simulink model "Aircraft6dof_V2"  (R2025b)
settings: Solver=ode4  StartTime=startTime  StopTime=A8.stopTime  FixedStep=stepTime  RelTol=1e-3  EnableMultiTasking=on
values from neighbouring files (symbols this model uses):
  A8 = struct()    [Setup_A8_master.m]
  InitAtt = InitAtt_deg * deg2rad    [Setup_A8_master.m]
  K_lqr_cmd = DeMixMatrix_val * K_lqr    [Design_LQR_Controller.m]
  n_p1 = axis_body    [Setup_A8_master.m]
undefined symbols (not defined in the file or in its folder): a0_s2, a0_s3, a0_s4, a0_s5, AR_s2, AR_s3, AR_s4, AR_s5, ARvecP1, Att_Trim, c_s2, c_s3, c_s4, c_s5, CD0_s2, CD0_s3, CD0_s4, CD0_s5, CDa_s2, CDa_s3, CDa_s4, CDa_s5, CL0_s2, CL0_s3, CL0_s4, CL0_s5, CM0_s2, CM0_s3, CM0_s4, CM0_s5, CMa_s2, CMa_s3, CMa_s4, CMa_s5, CQvecP1, CTvecP1, dCL_du, e_s2, e_s3, e_s4, e_s5, i_s2, i_s3, i_s4, i_s5, J, J_int, m, n_int, n_s2, n_s3, n_s4, n_s5, R_p1, Rates_Trim, S_s2, S_s3, S_s4, S_s5, S_u_s2 ... (+11)
libraries: vrlib x9, simulink x5
(part 2 of 3)

== system Aircraft6dof_V2/Actuators - Plant /AeroForcesAndMoments/Surface5 ==
  C_BW : Inport
  v_B_BA : Inport  Port=2
  rho : Inport  Port=3
  u_s#_rad : Inport  Port=4
  Constant : Constant  Value=n_s5
  Constant1 : Constant  Value=S_s5
  Constant10 : Constant  Value=CM0_s5
  Constant11 : Constant  Value=c_s5
  Constant12 : Constant  Value=x_s5
  Constant13 : Constant  Value=x_cm
  Constant15 : Constant  Value=S_u_s5
  Constant16 : Constant  Value=dCL_du
  Constant2 : Constant  Value=CD0_s5
  Constant3 : Constant  Value=i_s5
  Constant4 : Constant  Value=AR_s5
  Constant5 : Constant  Value=CL0_s5
  Constant6 : Constant  Value=CDa_s5
  Constant7 : Constant  Value=a0_s5
  Constant8 : Constant  Value=e_s5
  Constant9 : Constant  Value=CMa_s5
  Cross Product : vrlib/Utilities/Cross Product
  Display{,1..5} (6 alike) : Display
  Divide : Product  Inputs=/*
  Product : Product  Multiplication=Matrix(*)
  Subtract : Sum  Inputs=+-
  Subtract1 : Sum
  Surface# : Subsystem
  Fs5_B : Outport  VectorParamsAs1DForOutWhenUnconnected=off
  Ms5_B : Outport  Port=2  VectorParamsAs1DForOutWhenUnconnected=off
  wires:
  Constant8/1 -> Surface#/11(e_s#)
  Constant6/1 -> Surface#/9(CDa_s#)
  Constant2/1 -> Surface#/8(CD0_s#)
  rho/1 -> Surface#/6(rho)
  Constant5/1 -> Surface#/5(CL0_s#)
  Constant4/1 -> Surface#/4(AR_s#)
  Constant3/1 -> Surface#/3(i_s#)
  Constant/1 -> Surface#/2(n_s#)
  v_B_BA/1 -> Surface#/1(v_B_BA)
  Constant7/1 -> Surface#/10(a0_s#)
  Constant9/1 -> Surface#/12(CMa_s#)
  Constant11/1 -> Surface#/14(c_s#)
  Surface#/1(Fs#_W) -> Display/1, Product/2
  Constant10/1 -> Surface#/13(CM0_s#)
  Surface#/2(Ms#_B) -> Display1/1, Subtract1/2
  Subtract1/1 -> Display4/1, Ms5_B/1
  Product/1 -> Cross Product/2, Display3/1, Fs5_B/1
  Cross Product/1 -> Display2/1, Subtract1/1
  Constant13/1 -> Subtract/2
  Constant12/1 -> Subtract/1
  C_BW/1 -> Product/1
  Subtract/1 -> Cross Product/1, Display5/1
  Constant1/1 -> Surface#/7(S_s#), Divide/1
  u_s#_rad/1 -> Surface#/15(u_s#)
  Constant15/1 -> Divide/2
  Constant16/1 -> Surface#/17(dCL_du_s#)
  Divide/1 -> Surface#/16(Su_S_ratio_s#)

== system Aircraft6dof_V2/Actuators - Plant /Equations Of Motion State Equations/Earth Model ==
  p_E_E_BE : Inport
  Constant1 : Constant  Value=A8.init.Rearth
  Constant6 : Constant  Value=A8.init.g_E_N
  Terminator : Terminator
  Rearth : Outport  VectorParamsAs1DForOutWhenUnconnected=off
  g_N : Outport  Port=2  VectorParamsAs1DForOutWhenUnconnected=off
  wires:
  Constant6/1 -> g_N/1
  p_E_E_BE/1 -> Terminator/1
  Constant1/1 -> Rearth/1

== system Aircraft6dof_V2/Actuators - Plant /Equations Of Motion State Equations/QUAT2ATT ==
  q : Inport
  Mux : Mux  Inputs=3
  Trigonometric Function1 : Trigonometry  Operator=atan2
  Trigonometric Function3 : Trigonometry  Operator=atan2
  fcn1 : Fcn  Expr=2*(u[2]*u[3] + u[1]*u[4])
  fcn2 : Fcn  Expr=u[1]*u[1] + u[2]*u[2] - u[3]*u[3] - u[4]*u[4]
  fcn3 : Fcn  Expr=-2*(u[2]*u[4] - u[1]*u[3])
  fcn4 : Fcn  Expr=2*(u[3]*u[4] + u[1]*u[2])
  fcn5 : Fcn  Expr=u[1]*u[1] - u[2]*u[2] - u[3]*u[3] + u[4]*u[4]
  trigFcn : Trigonometry  Operator=asin
  ATT : Outport  VectorParamsAs1DForOutWhenUnconnected=off
  wires:
  q/1 -> fcn2/1, fcn1/1, fcn4/1, fcn5/1, fcn3/1
  Trigonometric Function3/1 -> Mux/1  "psi"
  trigFcn/1 -> Mux/2  "theta"
  Trigonometric Function1/1 -> Mux/3  "phi"
  Mux/1 -> ATT/1
  fcn3/1 -> trigFcn/1
  fcn1/1 -> Trigonometric Function1/1
  fcn2/1 -> Trigonometric Function1/2
  fcn4/1 -> Trigonometric Function3/1
  fcn5/1 -> Trigonometric Function3/2

== system Aircraft6dof_V2/Actuators - Plant /Equations Of Motion State Equations/QUAT2DCM ==
  Quat : Inport  PortDimensions=4
  Subsystem : Subsystem
  Subsystem1 : Subsystem
  Subsystem2 : Subsystem
  Subsystem3 : Subsystem
  Subsystem4 : Subsystem
  Subsystem5 : Subsystem
  Subsystem6 : Subsystem
  Subsystem7 : Subsystem
  Subsystem8 : Subsystem
  Vector Concatenate : Concatenate  NumInputs=3
  Vector Concatenate1 : Concatenate  NumInputs=3
  Vector Concatenate2 : Concatenate  NumInputs=3
  Vector Concatenate3 : Concatenate  NumInputs=3  Mode=Multidimensional array  ConcatenateDimension=2
  norm : Subsystem
  DCM : Outport  PortDimensions=[3,3]  InitialOutput=0  VectorParamsAs1DForOutWhenUnconnected=off
  wires:
  Subsystem1/1(A12) -> Vector Concatenate1/1
  Subsystem7/1(A22) -> Vector Concatenate1/2
  norm/1(q/|q|) -> Subsystem/1(normal(q)), Subsystem8/1(normal(q)), Subsystem4/1(normal(q)), Subsystem2/1(normal(q)), Subsystem6/1(normal(q)), Subsystem7/1(normal(q)), Subsystem1/1(normal(q)), Subsystem5/1(normal(q)), Subsystem3/1(normal(q))
  Quat/1 -> norm/1(q)
  Subsystem8/1(A33) -> Vector Concatenate2/3
  Subsystem4/1(A23) -> Vector Concatenate2/2
  Subsystem2/1(A13) -> Vector Concatenate2/1
  Subsystem6/1(A32) -> Vector Concatenate1/3
  Subsystem5/1(A31) -> Vector Concatenate/3
  Subsystem3/1(A21) -> Vector Concatenate/2
  Subsystem/1(A11) -> Vector Concatenate/1
  Vector Concatenate3/1 -> DCM/1
  Vector Concatenate/1 -> Vector Concatenate3/1
  Vector Concatenate1/1 -> Vector Concatenate3/2
  Vector Concatenate2/1 -> Vector Concatenate3/3

== system Aircraft6dof_V2/Actuators - Plant /Equations Of Motion State Equations/Rot Dyn (Moments) ==
  note: Old Internal rotational Component
      | New one is taken from Trim model
      | hx hy and hz are already included
      | Trim so we can just take the working
      | internal rot component block and use
      | its modified version
  Mext_B : Inport
  omDot_motor : Inport  Port=2
  Add : Sum  Inputs=+---
  Constant4 : Constant  Value=J
  Cross Product1 : vrlib/Utilities/Cross Product
  Integrate : Subsystem
  Internal Rotational Component 1 : Subsystem
  Internal Rotational Component 2 : Subsystem  Commented=on
  Product : Product  Multiplication=Matrix(*)
  Product1 : Product  Multiplication=Matrix(*)
  Scope : Scope
      settings: TimeSpan=100  ActiveDisplayYMinimum=-7.154E-26  ActiveDisplayYMaximum=-7.104E-26  DataLoggingVariableName=ScopeData14
  inv of matrix : MATLAB Function  TreatAsAtomicUnit=on
  om_B_B_BE : Outport  VectorParamsAs1DForOutWhenUnconnected=off
  om_motor : Outport  Port=2  VectorParamsAs1DForOutWhenUnconnected=off
  wires:
  Mext_B/1 -> Add/1
  Constant4/1 -> inv of matrix/1(u), Product/1
  Product/1 -> Cross Product1/2
  Cross Product1/1 -> Add/2
  inv of matrix/1(y) -> Product1/1
  Add/1 -> Product1/2
  omDot_motor/1 -> Internal Rotational Component 1/2(om_int_dot)
  Internal Rotational Component 1/1(hInt) -> Add/3
  Internal Rotational Component 1/2(hIntDot) -> Add/4
  Internal Rotational Component 1/3(om_motor) -> om_motor/1
  Integrate/1(om) -> Scope/1, Internal Rotational Component 1/1(om_B_B_BE), Cross Product1/1, Product/2, om_B_B_BE/1
  Product1/1 -> Integrate/1(omDot)

== system Aircraft6dof_V2/Actuators - Plant /Equations Of Motion State Equations/Rot Kin (Orientation) Euler ==
  om_B_B_BN : Inport
  Integrate : Subsystem
  MATLAB Function : MATLAB Function  TreatAsAtomicUnit=on
  Product : Product  Multiplication=Matrix(*)
  ATT_BN : Outport  VectorParamsAs1DForOutWhenUnconnected=off
  wires:
  om_B_B_BN/1 -> Product/2
  Product/1 -> Integrate/1(AttDot)
  Integrate/1(Att) -> MATLAB Function/1(ATT), ATT_BN/1
  MATLAB Function/1(MATRIX) -> Product/1

== system Aircraft6dof_V2/Actuators - Plant /Equations Of Motion State Equations/Rot Kin (Orientation) Quaternion ==
  om_B_B_BN : Inport
  Constant1 : Constant  Value=0
  Constant2 : Constant  Value=A8.init.InitQuat
  Demux : Demux  Outputs=3
  Gain : Gain  Gain=1/2
  Mux : Mux
  QuatMult : Subsystem
  QuatStates : Integrator  InitialConditionSource=external
  norm1 : Subsystem
  q_BN : Outport  VectorParamsAs1DForOutWhenUnconnected=off
  wires:
  Constant2/1 -> QuatStates/2
  om_B_B_BN/1 -> Demux/1
  Demux/3 -> Mux/4
  Demux/2 -> Mux/3
  Demux/1 -> Mux/2
  Constant1/1 -> Mux/1
  Mux/1 -> QuatMult/2(r)
  QuatMult/1(q*r) -> Gain/1
  Gain/1 -> QuatStates/1
  QuatStates/1 -> norm1/1(q)
  norm1/1(q/|q|) -> QuatMult/1(q), q_BN/1

== system Aircraft6dof_V2/Actuators - Plant /Equations Of Motion State Equations/Trans Dyn (Forces) ==
  Fext_B : Inport
  g_B : Inport  Port=2
  om_B_B_BE : Inport  Port=3
  Add : Sum  Inputs=++-
  Constant4 : Constant  Value=m
  Cross Product : vrlib/Utilities/Cross Product
  Display{,1..4} (5 alike) : Display
  Divide2 : Product  Inputs=*/
  Integrate : Subsystem
  xDot_E_B_BE : Outport  VectorParamsAs1DForOutWhenUnconnected=off
  accelMeasCG : Outport  Port=2  VectorParamsAs1DForOutWhenUnconnected=off
  wires:
  Add/1 -> Integrate/1(VelDot), Display/1  "xDotDot_E_B_BE"
  g_B/1 -> Display3/1, Add/2  "g_B"
  Fext_B/1 -> Divide2/1
  Constant4/1 -> Divide2/2
  Divide2/1 -> accelMeasCG/1, Display2/1, Add/1
  om_B_B_BE/1 -> Cross Product/1
  Integrate/1(Vel) -> Cross Product/2, Display1/1, xDot_E_B_BE/1
  Cross Product/1 -> Display4/1, Add/3

== system Aircraft6dof_V2/Actuators - Plant /Equations Of Motion State Equations/Trans Kin (Spherical) ==
  v_E_B_BE : Inport
  C_NB : Inport  Port=2
  Rearth : Inport  Port=3
  AltDot : Gain  Gain=-1
  Constant2 : Constant  Value=A8.init.InitPos
  Demux : Demux  Outputs=3
  Demux1 : Demux  Outputs=3
  Demux2 : Demux  Outputs=3
  LatDot : Subsystem
  LonDot : Subsystem
  Mux : Mux  Inputs=3
  Mux1 : Mux  Inputs=3
  PositionStates : Integrator  InitialConditionSource=external
  Product : Product  Multiplication=Matrix(*)
  Terminator : Terminator
  bound lat : Saturate  UpperLimit=pi/2  LowerLimit=-pi/2
  wrap lon : Subsystem
  p_E_E_BE : Outport  VectorParamsAs1DForOutWhenUnconnected=off
  wires:
  Mux1/1 -> p_E_E_BE/1, Demux1/1
  Product/1 -> Demux/1
  Rearth/1 -> LatDot/2(Rearth), LonDot/2(Rearth)
  Demux1/3 -> LatDot/3(alt), LonDot/3(alt)
  Demux/3 -> AltDot/1
  AltDot/1 -> Mux/3
  Mux/1 -> PositionStates/1
  Constant2/1 -> PositionStates/2
  Demux1/2 -> Terminator/1
  PositionStates/1 -> Demux2/1
  Demux2/1 -> bound lat/1
  bound lat/1 -> Mux1/1
  Demux2/3 -> Mux1/3
  Demux2/2 -> wrap lon/1(lon)
  wrap lon/1(-pi < lon <= pi) -> Mux1/2
  C_NB/1 -> Product/1
  v_E_B_BE/1 -> Product/2
  Demux/1 -> LatDot/1(Vn)
  LatDot/1(latDot) -> Mux/1
  Demux/2 -> LonDot/1(Ve)
  Demux1/1 -> LonDot/4(lat)
  LonDot/1(lonDot) -> Mux/2

== system Aircraft6dof_V2/Actuators - Plant /PropulsionForcesAndMoments/PropulsionSystem1 ==
  Om_p1 : Inport
  v_B_BA : Inport  Port=2
  rho : Inport  Port=3
  u_p#_pct : Inport  Port=4
  Constant : Constant  Value=n_p1
  Constant1 : Constant  Value=A8.init.battery.nCellsSeries
  Constant11 : Constant  Value=R_p1
  Constant12 : Constant  Value=x_p1
  Constant13 : Constant  Value=x_cm
  Constant2 : Constant  Value=A8.init.battery.VcellMax
  Constant3 : Constant  Value=A8.init.motor.Rmotor
  Constant4 : Constant  Value=A8.init.motor.Io_motor
  Constant5 : Constant  Value=A8.init.motor.Ki_motor
  Constant6 : Constant  Value=A8.init.motor.J_int(1)
  Cross Product : vrlib/Utilities/Cross Product
  Display{,1..5} (6 alike) : Display
  PropulstionSystem# : Subsystem
  Subtract : Sum  Inputs=+-
  Subtract1 : Sum
  Fs4_B : Outport  VectorParamsAs1DForOutWhenUnconnected=off
  Ms4_B : Outport  Port=2  VectorParamsAs1DForOutWhenUnconnected=off
  omDot : Outport  Port=3  VectorParamsAs1DForOutWhenUnconnected=off
  wires:
  u_p#_pct/1 -> PropulstionSystem#/6(u_s#)
  rho/1 -> PropulstionSystem#/4(rho)
  Constant/1 -> PropulstionSystem#/2(n_p#)
  v_B_BA/1 -> PropulstionSystem#/1(v_B_BA)
  Constant11/1 -> PropulstionSystem#/5(R_p#)
  PropulstionSystem#/2(Mp#_B) -> Display1/1, Subtract1/2
  Subtract1/1 -> Display4/1, Ms4_B/1
  PropulstionSystem#/1(Fp#_B) -> Display/1, Cross Product/2, Display3/1, Fs4_B/1
  Cross Product/1 -> Subtract1/1, Display2/1
  Constant13/1 -> Subtract/2
  Constant12/1 -> Subtract/1
  Subtract/1 -> Cross Product/1, Display5/1
  Om_p1/1 -> PropulstionSystem#/3(Om_p#)
  Constant1/1 -> PropulstionSystem#/7(nCellsSeries)
  Constant2/1 -> PropulstionSystem#/8(VcallMax)
  Constant3/1 -> PropulstionSystem#/9(Rmotor)
  Constant4/1 -> PropulstionSystem#/10(Io_motor)
  Constant5/1 -> PropulstionSystem#/11(Ki_motor)
  Constant6/1 -> PropulstionSystem#/12(J_p1)
  PropulstionSystem#/3(omDot_Motor) -> omDot/1

== system Aircraft6dof_V2/Controller/PID Controller/wrap hdg ==
  hdg_err : Inport
  Add : Sum  Inputs=-+
  Add1 : Sum
  Compare To Constant : simulink/Logic and Bit Operations/Compare To Constant  relop=>  const=pi  OutDataTypeStr=boolean
  Compare To Constant1 : simulink/Logic and Bit Operations/Compare To Constant  relop=<=  const=-pi  OutDataTypeStr=boolean
  Constant : Constant  Value=2*pi
  Switch : Switch  Criteria=u2 > Threshold  SaturateOnIntegerOverflow=off  InputSameDT=off
  Switch1 : Switch  Criteria=u2 > Threshold  SaturateOnIntegerOverflow=off  InputSameDT=off
  <+/-pi : Outport  VectorParamsAs1DForOutWhenUnconnected=off
  wires:
  hdg_err/1 -> Compare To Constant/1, Add/2, Switch/3
  Add/1 -> Switch/1
  Compare To Constant/1 -> Switch/2
  Compare To Constant1/1 -> Switch1/2
  Switch/1 -> Switch1/3, Add1/2, Compare To Constant1/1
  Switch1/1 -> <+/-pi/1
  Constant/1 -> Add/1, Add1/1
  Add1/1 -> Switch1/1

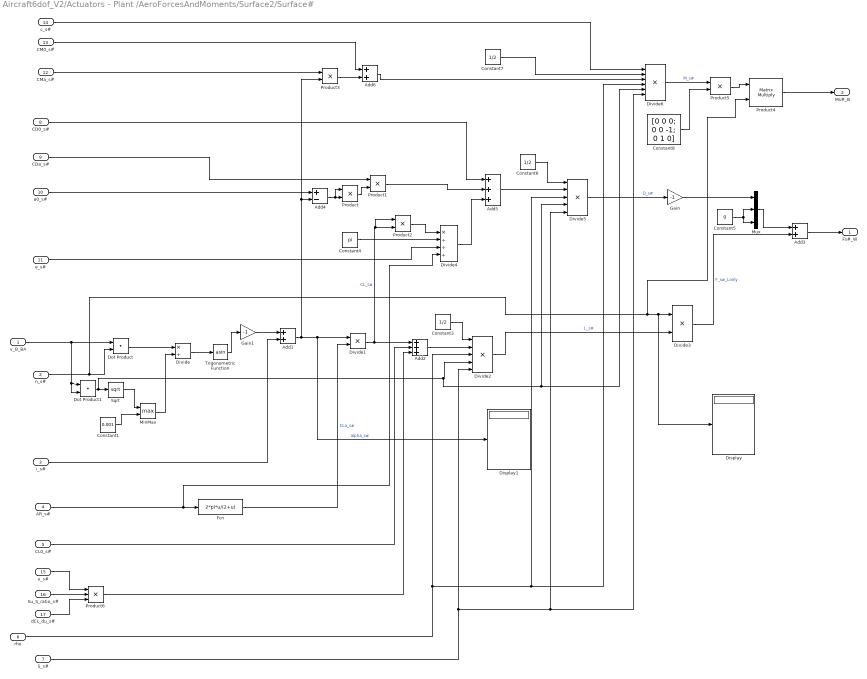
== system Aircraft6dof_V2/Actuators - Plant /AeroForcesAndMoments/Surface2/Surface# ==
  v_B_BA : Inport
  n_s# : Inport  Port=2
  i_s# : Inport  Port=3
  AR_s# : Inport  Port=4
  CL0_s# : Inport  Port=5
  rho : Inport  Port=6
  S_s# : Inport  Port=7
  CD0_s# : Inport  Port=8
  CDa_s# : Inport  Port=9
  a0_s# : Inport  Port=10
  e_s# : Inport  Port=11
  CMa_s# : Inport  Port=12
  CM0_s# : Inport  Port=13
  c_s# : Inport  Port=14
  u_s# : Inport  Port=15
  Su_S_ratio_s# : Inport  Port=16
  dCL_du_s# : Inport  Port=17
  Add1 : Sum
  Add2 : Sum  Inputs=+++
  Add3 : Sum
  Add4 : Sum  Inputs=+-
  Add5 : Sum  Inputs=+++
  Add6 : Sum
  Constant1 : Constant  Value=0.001
  Constant3 : Constant  Value=1/2
  Constant4 : Constant  Value=pi
  Constant5 : Constant  Value=0
  Constant6 : Constant  Value=1/2
  Constant7 : Constant  Value=1/2
  Constant8 : Constant  Value=[0 0 0; 0 0 -1; 0 1 0]
  Display : Display
  Display1 : Display
  Divide : Product  Inputs=*/
  Divide1 : Product  Inputs=**
  Divide2 : Product  Inputs=*****
  Divide3 : Product  Inputs=**
  Divide4 : Product  Inputs=*///
  Divide5 : Product  Inputs=*****
  Divide6 : Product  Inputs=******
  Dot Product : DotProduct  OutDataTypeStr=Inherit: Inherit via internal rule
  Dot Product1 : DotProduct  OutDataTypeStr=Inherit: Inherit via internal rule
  Fcn : Fcn  Expr=2*pi*u/(2+u)
  Gain : Gain  Gain=-1
  Gain1 : Gain  Gain=-1
  MinMax : MinMax  Function=max  Inputs=2
  Mux : Mux  Inputs=3
  Product{,1..3,5} (5 alike) : Product
  Product4 : Product  Multiplication=Matrix(*)
  Product6 : Product  Inputs=3
  Sqrt : Sqrt
  Trigonometric Function : Trigonometry  Operator=asin
  Fs#_W : Outport  VectorParamsAs1DForOutWhenUnconnected=off
  Ms#_B : Outport  Port=2  VectorParamsAs1DForOutWhenUnconnected=off
  wires:
  v_B_BA/1 -> Dot Product1/1, Dot Product1/2, Dot Product/1
  n_s#/1 -> Product4/2, Display/1, Divide3/1, Dot Product/2
  Dot Product/1 -> Divide/1
  Constant1/1 -> MinMax/2
  MinMax/1 -> Divide/2
  Sqrt/1 -> MinMax/1
  Divide/1 -> Trigonometric Function/1
  i_s#/1 -> Add1/2
  Add1/1 -> Product3/2, Add4/2, Display1/1, Divide1/1  "alpha_s#"
  AR_s#/1 -> Divide4/4, Fcn/1
  Fcn/1 -> Divide1/2  "CLa_s#"
  Divide1/1 -> Product2/1, Product2/2, Add2/1  "CL_s#"
  CL0_s#/1 -> Add2/2
  Add2/1 -> Divide2/2
  Constant3/1 -> Divide2/1
  Divide2/1 -> Divide3/2  "L_s#"
  Divide3/1 -> Add3/2  "F_s#_Lonly"
  Mux/1 -> Add3/1
  a0_s#/1 -> Add4/1
  Add4/1 -> Product/1, Product/2
  Product/1 -> Product1/2
  CDa_s#/1 -> Product1/1
  Product2/1 -> Divide4/1
  Constant4/1 -> Divide4/2
  e_s#/1 -> Divide4/3
  Divide4/1 -> Add5/3
  Product1/1 -> Add5/2
  CD0_s#/1 -> Add5/1
  Add5/1 -> Divide5/2
  Constant5/1 -> Mux/2, Mux/3
  CMa_s#/1 -> Product3/1
  CM0_s#/1 -> Add6/1
  Product3/1 -> Add6/2
  Constant6/1 -> Divide5/1
  Divide5/1 -> Gain/1  "D_s#"
  Dot Product1/1 -> Divide6/5, Divide5/4, Divide2/4, Sqrt/1
  rho/1 -> Divide6/4, Divide5/3, Divide2/3
  S_s#/1 -> Divide6/6, Divide5/5, Divide2/5
  Add6/1 -> Divide6/3
  Constant7/1 -> Divide6/2
  c_s#/1 -> Divide6/1
  Add3/1 -> Fs#_W/1
  Divide6/1 -> Product5/1  "M_s#"
  Constant8/1 -> Product5/2
  Product4/1 -> Ms#_B/1
  Product5/1 -> Product4/1
  Gain/1 -> Mux/1
  Gain1/1 -> Add1/1
  Trigonometric Function/1 -> Gain1/1
  u_s#/1 -> Product6/1
  Su_S_ratio_s#/1 -> Product6/2
  dCL_du_s#/1 -> Product6/3
  Product6/1 -> Add2/3

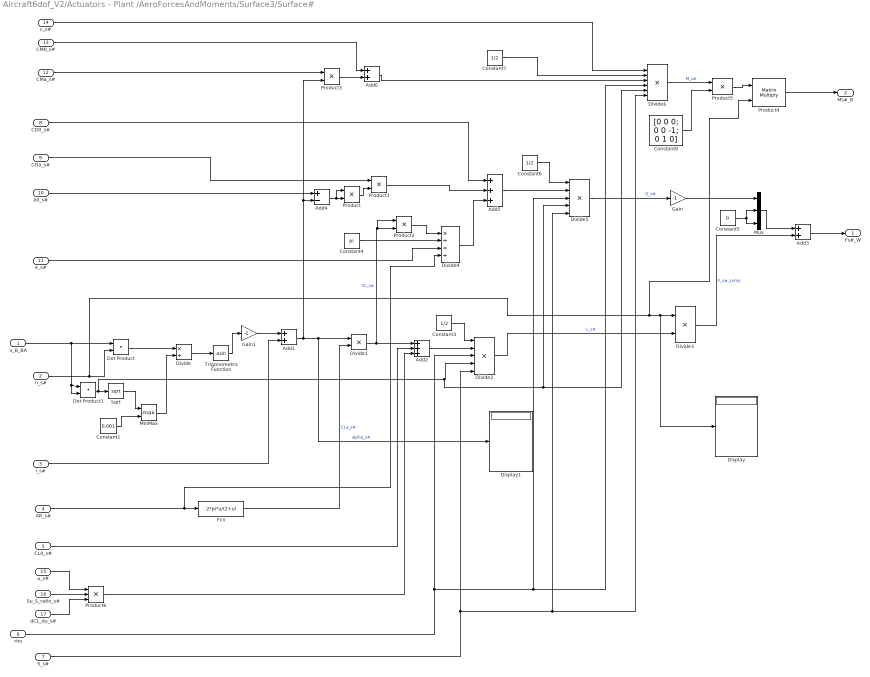
== system Aircraft6dof_V2/Actuators - Plant /AeroForcesAndMoments/Surface3/Surface# ==
  v_B_BA : Inport
  n_s# : Inport  Port=2
  i_s# : Inport  Port=3
  AR_s# : Inport  Port=4
  CL0_s# : Inport  Port=5
  rho : Inport  Port=6
  S_s# : Inport  Port=7
  CD0_s# : Inport  Port=8
  CDa_s# : Inport  Port=9
  a0_s# : Inport  Port=10
  e_s# : Inport  Port=11
  CMa_s# : Inport  Port=12
  CM0_s# : Inport  Port=13
  c_s# : Inport  Port=14
  u_s# : Inport  Port=15
  Su_S_ratio_s# : Inport  Port=16
  dCL_du_s# : Inport  Port=17
  Add1 : Sum
  Add2 : Sum  Inputs=+++
  Add3 : Sum
  Add4 : Sum  Inputs=+-
  Add5 : Sum  Inputs=+++
  Add6 : Sum
  Constant1 : Constant  Value=0.001
  Constant3 : Constant  Value=1/2
  Constant4 : Constant  Value=pi
  Constant5 : Constant  Value=0
  Constant6 : Constant  Value=1/2
  Constant7 : Constant  Value=1/2
  Constant8 : Constant  Value=[0 0 0; 0 0 -1; 0 1 0]
  Display : Display
  Display1 : Display
  Divide : Product  Inputs=*/
  Divide1 : Product  Inputs=**
  Divide2 : Product  Inputs=*****
  Divide3 : Product  Inputs=**
  Divide4 : Product  Inputs=*///
  Divide5 : Product  Inputs=*****
  Divide6 : Product  Inputs=******
  Dot Product : DotProduct  OutDataTypeStr=Inherit: Inherit via internal rule
  Dot Product1 : DotProduct  OutDataTypeStr=Inherit: Inherit via internal rule
  Fcn : Fcn  Expr=2*pi*u/(2+u)
  Gain : Gain  Gain=-1
  Gain1 : Gain  Gain=-1
  MinMax : MinMax  Function=max  Inputs=2
  Mux : Mux  Inputs=3
  Product{,1..3,5} (5 alike) : Product
  Product4 : Product  Multiplication=Matrix(*)
  Product6 : Product  Inputs=3
  Sqrt : Sqrt
  Trigonometric Function : Trigonometry  Operator=asin
  Fs#_W : Outport  VectorParamsAs1DForOutWhenUnconnected=off
  Ms#_B : Outport  Port=2  VectorParamsAs1DForOutWhenUnconnected=off
  wires:
  v_B_BA/1 -> Dot Product1/1, Dot Product1/2, Dot Product/1
  n_s#/1 -> Product4/2, Display/1, Divide3/1, Dot Product/2
  Dot Product/1 -> Divide/1
  Constant1/1 -> MinMax/2
  MinMax/1 -> Divide/2
  Sqrt/1 -> MinMax/1
  Divide/1 -> Trigonometric Function/1
  i_s#/1 -> Add1/2
  Add1/1 -> Product3/2, Add4/2, Display1/1, Divide1/1  "alpha_s#"
  AR_s#/1 -> Divide4/4, Fcn/1
  Fcn/1 -> Divide1/2  "CLa_s#"
  Divide1/1 -> Product2/1, Product2/2, Add2/1  "CL_s#"
  CL0_s#/1 -> Add2/2
  Add2/1 -> Divide2/2
  Constant3/1 -> Divide2/1
  Divide2/1 -> Divide3/2  "L_s#"
  Divide3/1 -> Add3/2  "F_s#_Lonly"
  Mux/1 -> Add3/1
  a0_s#/1 -> Add4/1
  Add4/1 -> Product/1, Product/2
  Product/1 -> Product1/2
  CDa_s#/1 -> Product1/1
  Product2/1 -> Divide4/1
  Constant4/1 -> Divide4/2
  e_s#/1 -> Divide4/3
  Divide4/1 -> Add5/3
  Product1/1 -> Add5/2
  CD0_s#/1 -> Add5/1
  Add5/1 -> Divide5/2
  Constant5/1 -> Mux/2, Mux/3
  CMa_s#/1 -> Product3/1
  CM0_s#/1 -> Add6/1
  Product3/1 -> Add6/2
  Constant6/1 -> Divide5/1
  Divide5/1 -> Gain/1  "D_s#"
  Dot Product1/1 -> Divide6/5, Divide5/4, Divide2/4, Sqrt/1
  rho/1 -> Divide6/4, Divide5/3, Divide2/3
  S_s#/1 -> Divide6/6, Divide5/5, Divide2/5
  Add6/1 -> Divide6/3
  Constant7/1 -> Divide6/2
  c_s#/1 -> Divide6/1
  Add3/1 -> Fs#_W/1
  Divide6/1 -> Product5/1  "M_s#"
  Constant8/1 -> Product5/2
  Product4/1 -> Ms#_B/1
  Product5/1 -> Product4/1
  Gain/1 -> Mux/1
  Gain1/1 -> Add1/1
  Trigonometric Function/1 -> Gain1/1
  u_s#/1 -> Product6/1
  Su_S_ratio_s#/1 -> Product6/2
  dCL_du_s#/1 -> Product6/3
  Product6/1 -> Add2/3

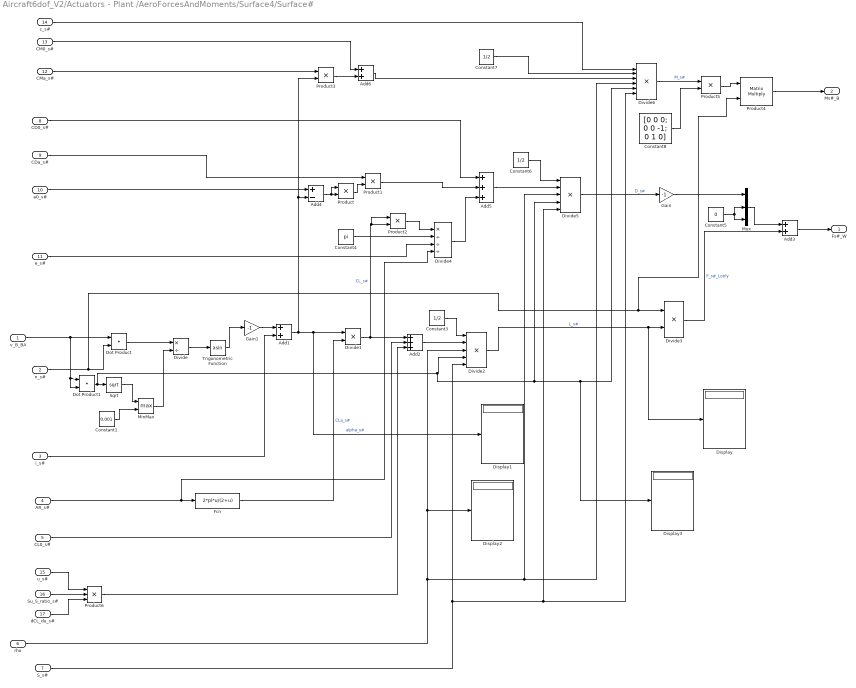
== system Aircraft6dof_V2/Actuators - Plant /AeroForcesAndMoments/Surface4/Surface# ==
  v_B_BA : Inport
  n_s# : Inport  Port=2
  i_s# : Inport  Port=3
  AR_s# : Inport  Port=4
  CL0_s# : Inport  Port=5
  rho : Inport  Port=6
  S_s# : Inport  Port=7
  CD0_s# : Inport  Port=8
  CDa_s# : Inport  Port=9
  a0_s# : Inport  Port=10
  e_s# : Inport  Port=11
  CMa_s# : Inport  Port=12
  CM0_s# : Inport  Port=13
  c_s# : Inport  Port=14
  u_s# : Inport  Port=15
  Su_S_ratio_s# : Inport  Port=16
  dCL_du_s# : Inport  Port=17
  Add1 : Sum
  Add2 : Sum  Inputs=+++
  Add3 : Sum
  Add4 : Sum  Inputs=+-
  Add5 : Sum  Inputs=+++
  Add6 : Sum
  Constant1 : Constant  Value=0.001
  Constant3 : Constant  Value=1/2
  Constant4 : Constant  Value=pi
  Constant5 : Constant  Value=0
  Constant6 : Constant  Value=1/2
  Constant7 : Constant  Value=1/2
  Constant8 : Constant  Value=[0 0 0; 0 0 -1; 0 1 0]
  Display{,1..3} (4 alike) : Display
  Divide : Product  Inputs=*/
  Divide1 : Product  Inputs=**
  Divide2 : Product  Inputs=*****
  Divide3 : Product  Inputs=**
  Divide4 : Product  Inputs=*///
  Divide5 : Product  Inputs=*****
  Divide6 : Product  Inputs=******
  Dot Product : DotProduct  OutDataTypeStr=Inherit: Inherit via internal rule
  Dot Product1 : DotProduct  OutDataTypeStr=Inherit: Inherit via internal rule
  Fcn : Fcn  Expr=2*pi*u/(2+u)
  Gain : Gain  Gain=-1
  Gain1 : Gain  Gain=-1
  MinMax : MinMax  Function=max  Inputs=2
  Mux : Mux  Inputs=3
  Product{,1..3,5} (5 alike) : Product
  Product4 : Product  Multiplication=Matrix(*)
  Product6 : Product  Inputs=3
  Sqrt : Sqrt
  Trigonometric Function : Trigonometry  Operator=asin
  Fs#_W : Outport  VectorParamsAs1DForOutWhenUnconnected=off
  Ms#_B : Outport  Port=2  VectorParamsAs1DForOutWhenUnconnected=off
  wires:
  v_B_BA/1 -> Dot Product1/1, Dot Product1/2, Dot Product/1
  n_s#/1 -> Product4/2, Divide3/1, Dot Product/2
  Dot Product/1 -> Divide/1
  Constant1/1 -> MinMax/2
  MinMax/1 -> Divide/2
  Sqrt/1 -> MinMax/1
  Divide/1 -> Trigonometric Function/1
  Gain1/1 -> Add1/1
  i_s#/1 -> Add1/2
  Add1/1 -> Product3/2, Add4/2, Display1/1, Divide1/1  "alpha_s#"
  AR_s#/1 -> Divide4/4, Fcn/1
  Fcn/1 -> Divide1/2  "CLa_s#"
  Divide1/1 -> Product2/1, Product2/2, Add2/1  "CL_s#"
  CL0_s#/1 -> Add2/2
  Add2/1 -> Divide2/2
  Constant3/1 -> Divide2/1
  Divide2/1 -> Display/1, Divide3/2  "L_s#"
  Divide3/1 -> Add3/2  "F_s#_Lonly"
  Mux/1 -> Add3/1
  a0_s#/1 -> Add4/1
  Add4/1 -> Product/1, Product/2
  Product/1 -> Product1/2
  CDa_s#/1 -> Product1/1
  Product2/1 -> Divide4/1
  Constant4/1 -> Divide4/2
  e_s#/1 -> Divide4/3
  Divide4/1 -> Add5/3
  Product1/1 -> Add5/2
  CD0_s#/1 -> Add5/1
  Add5/1 -> Divide5/2
  Constant5/1 -> Mux/2, Mux/3
  CMa_s#/1 -> Product3/1
  CM0_s#/1 -> Add6/1
  Product3/1 -> Add6/2
  Constant6/1 -> Divide5/1
  Divide5/1 -> Gain/1  "D_s#"
  Dot Product1/1 -> Display3/1, Divide6/5, Divide5/4, Divide2/4, Sqrt/1
  rho/1 -> Divide6/4, Divide5/3, Display2/1, Divide2/3
  S_s#/1 -> Divide6/6, Divide5/5, Divide2/5
  Add6/1 -> Divide6/3
  Constant7/1 -> Divide6/2
  c_s#/1 -> Divide6/1
  Add3/1 -> Fs#_W/1
  Divide6/1 -> Product5/1  "M_s#"
  Constant8/1 -> Product5/2
  Product4/1 -> Ms#_B/1
  Product5/1 -> Product4/1
  Gain/1 -> Mux/1
  Trigonometric Function/1 -> Gain1/1
  u_s#/1 -> Product6/1
  Su_S_ratio_s#/1 -> Product6/2
  dCL_du_s#/1 -> Product6/3
  Product6/1 -> Add2/3

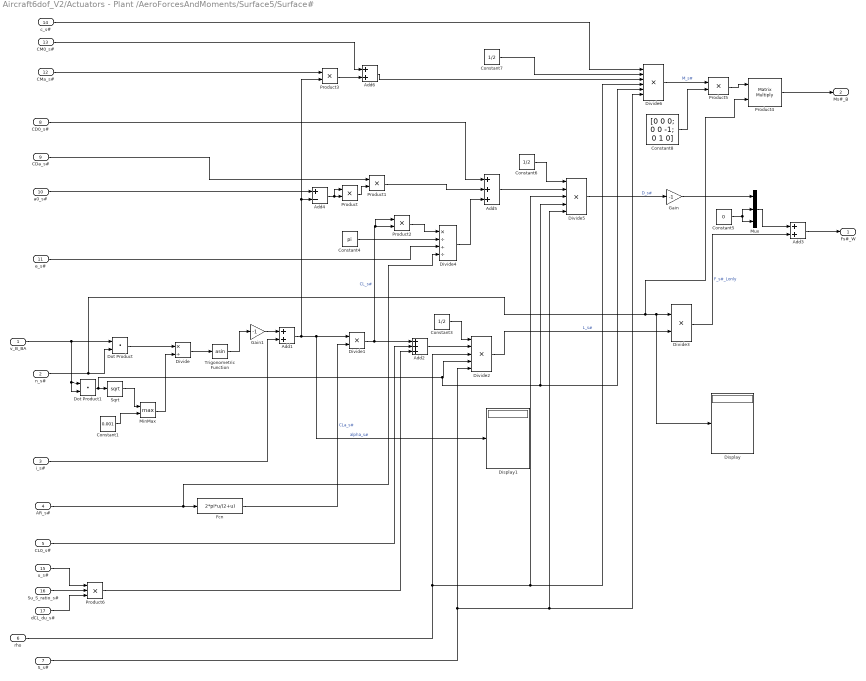
== system Aircraft6dof_V2/Actuators - Plant /AeroForcesAndMoments/Surface5/Surface# ==
  v_B_BA : Inport
  n_s# : Inport  Port=2
  i_s# : Inport  Port=3
  AR_s# : Inport  Port=4
  CL0_s# : Inport  Port=5
  rho : Inport  Port=6
  S_s# : Inport  Port=7
  CD0_s# : Inport  Port=8
  CDa_s# : Inport  Port=9
  a0_s# : Inport  Port=10
  e_s# : Inport  Port=11
  CMa_s# : Inport  Port=12
  CM0_s# : Inport  Port=13
  c_s# : Inport  Port=14
  u_s# : Inport  Port=15
  Su_S_ratio_s# : Inport  Port=16
  dCL_du_s# : Inport  Port=17
  Add1 : Sum
  Add2 : Sum  Inputs=+++
  Add3 : Sum
  Add4 : Sum  Inputs=+-
  Add5 : Sum  Inputs=+++
  Add6 : Sum
  Constant1 : Constant  Value=0.001
  Constant3 : Constant  Value=1/2
  Constant4 : Constant  Value=pi
  Constant5 : Constant  Value=0
  Constant6 : Constant  Value=1/2
  Constant7 : Constant  Value=1/2
  Constant8 : Constant  Value=[0 0 0; 0 0 -1; 0 1 0]
  Display : Display
  Display1 : Display
  Divide : Product  Inputs=*/
  Divide1 : Product  Inputs=**
  Divide2 : Product  Inputs=*****
  Divide3 : Product  Inputs=**
  Divide4 : Product  Inputs=*///
  Divide5 : Product  Inputs=*****
  Divide6 : Product  Inputs=******
  Dot Product : DotProduct  OutDataTypeStr=Inherit: Inherit via internal rule
  Dot Product1 : DotProduct  OutDataTypeStr=Inherit: Inherit via internal rule
  Fcn : Fcn  Expr=2*pi*u/(2+u)
  Gain : Gain  Gain=-1
  Gain1 : Gain  Gain=-1
  MinMax : MinMax  Function=max  Inputs=2
  Mux : Mux  Inputs=3
  Product{,1..3,5} (5 alike) : Product
  Product4 : Product  Multiplication=Matrix(*)
  Product6 : Product  Inputs=3
  Sqrt : Sqrt
  Trigonometric Function : Trigonometry  Operator=asin
  Fs#_W : Outport  VectorParamsAs1DForOutWhenUnconnected=off
  Ms#_B : Outport  Port=2  VectorParamsAs1DForOutWhenUnconnected=off
  wires:
  Gain/1 -> Mux/1
  Product5/1 -> Product4/1
  Product4/1 -> Ms#_B/1
  Constant8/1 -> Product5/2
  Divide6/1 -> Product5/1  "M_s#"
  Add3/1 -> Fs#_W/1
  c_s#/1 -> Divide6/1
  Constant7/1 -> Divide6/2
  Add6/1 -> Divide6/3
  S_s#/1 -> Divide2/5, Divide5/5, Divide6/6
  rho/1 -> Divide2/3, Divide5/3, Divide6/4
  Dot Product1/1 -> Sqrt/1, Divide2/4, Divide5/4, Divide6/5
  Divide5/1 -> Gain/1  "D_s#"
  Constant6/1 -> Divide5/1
  Product3/1 -> Add6/2
  CM0_s#/1 -> Add6/1
  CMa_s#/1 -> Product3/1
  Constant5/1 -> Mux/3, Mux/2
  Add5/1 -> Divide5/2
  CD0_s#/1 -> Add5/1
  Product1/1 -> Add5/2
  Divide4/1 -> Add5/3
  e_s#/1 -> Divide4/3
  Constant4/1 -> Divide4/2
  Product2/1 -> Divide4/1
  CDa_s#/1 -> Product1/1
  Product/1 -> Product1/2
  Add4/1 -> Product/2, Product/1
  a0_s#/1 -> Add4/1
  Mux/1 -> Add3/1
  Divide3/1 -> Add3/2  "F_s#_Lonly"
  Divide2/1 -> Divide3/2  "L_s#"
  Constant3/1 -> Divide2/1
  Add2/1 -> Divide2/2
  CL0_s#/1 -> Add2/2
  Divide1/1 -> Add2/1, Product2/2, Product2/1  "CL_s#"
  Fcn/1 -> Divide1/2  "CLa_s#"
  AR_s#/1 -> Fcn/1, Divide4/4
  Add1/1 -> Divide1/1, Display1/1, Add4/2, Product3/2  "alpha_s#"
  i_s#/1 -> Add1/2
  Divide/1 -> Trigonometric Function/1
  Sqrt/1 -> MinMax/1
  MinMax/1 -> Divide/2
  Constant1/1 -> MinMax/2
  Dot Product/1 -> Divide/1
  n_s#/1 -> Dot Product/2, Divide3/1, Display/1, Product4/2
  v_B_BA/1 -> Dot Product/1, Dot Product1/2, Dot Product1/1
  Gain1/1 -> Add1/1
  Trigonometric Function/1 -> Gain1/1
  u_s#/1 -> Product6/1
  Su_S_ratio_s#/1 -> Product6/2
  dCL_du_s#/1 -> Product6/3
  Product6/1 -> Add2/3

== system Aircraft6dof_V2/Actuators - Plant /Equations Of Motion State Equations/QUAT2DCM/Subsystem ==
  normal(q) : Inport
  Demux : Demux
  Product{,1..3} (4 alike) : Product  RndMeth=Zero
  Sum : Sum  Inputs=++--
  A11 : Outport  VectorParamsAs1DForOutWhenUnconnected=off
  wires:
  Product3/1 -> Sum/1
  Demux/2 -> Product2/2, Product2/1
  Product1/1 -> Sum/3
  Demux/3 -> Product1/2, Product1/1
  Product2/1 -> Sum/2
  Sum/1 -> A11/1
  Product/1 -> Sum/4
  Demux/1 -> Product3/2, Product3/1
  normal(q)/1 -> Demux/1
  Demux/4 -> Product/2, Product/1

== system Aircraft6dof_V2/Actuators - Plant /Equations Of Motion State Equations/QUAT2DCM/Subsystem1 ==
  normal(q) : Inport
  Demux : Demux
  Gain : Gain  Gain=2
  Product2 : Product  RndMeth=Zero
  Product3 : Product  RndMeth=Zero
  Sum : Sum  Inputs=|++
  A12 : Outport  VectorParamsAs1DForOutWhenUnconnected=off
  wires:
  Product2/1 -> Sum/2
  Product3/1 -> Sum/1
  Sum/1 -> Gain/1
  Demux/1 -> Product3/2
  Demux/2 -> Product2/1
  Demux/4 -> Product3/1
  Demux/3 -> Product2/2
  normal(q)/1 -> Demux/1
  Gain/1 -> A12/1

== system Aircraft6dof_V2/Actuators - Plant /Equations Of Motion State Equations/QUAT2DCM/Subsystem2 ==
  normal(q) : Inport
  Demux : Demux
  Gain : Gain  Gain=2
  Product1 : Product  RndMeth=Zero
  Product2 : Product  RndMeth=Zero
  Sum : Sum  Inputs=|-+
  A13 : Outport  VectorParamsAs1DForOutWhenUnconnected=off
  wires:
  Demux/1 -> Product1/1
  Product1/1 -> Sum/1
  Product2/1 -> Sum/2
  Demux/4 -> Product2/2
  Demux/2 -> Product2/1
  Demux/3 -> Product1/2
  normal(q)/1 -> Demux/1
  Gain/1 -> A13/1
  Sum/1 -> Gain/1

== system Aircraft6dof_V2/Actuators - Plant /Equations Of Motion State Equations/QUAT2DCM/Subsystem3 ==
  normal(q) : Inport
  Demux : Demux
  Gain : Gain  Gain=2
  Product2 : Product  RndMeth=Zero
  Product3 : Product  RndMeth=Zero
  Sum : Sum  Inputs=|-+
  A21 : Outport  VectorParamsAs1DForOutWhenUnconnected=off
  wires:
  Gain/1 -> A21/1
  normal(q)/1 -> Demux/1
  Demux/3 -> Product2/2
  Demux/4 -> Product3/1
  Demux/2 -> Product2/1
  Demux/1 -> Product3/2
  Sum/1 -> Gain/1
  Product3/1 -> Sum/1
  Product2/1 -> Sum/2

== system Aircraft6dof_V2/Actuators - Plant /Equations Of Motion State Equations/QUAT2DCM/Subsystem4 ==
  normal(q) : Inport
  Demux : Demux
  Gain : Gain  Gain=2
  Product1 : Product  RndMeth=Zero
  Product2 : Product  RndMeth=Zero
  Sum : Sum  Inputs=|++
  A23 : Outport  VectorParamsAs1DForOutWhenUnconnected=off
  wires:
  Demux/4 -> Product2/2
  Product2/1 -> Sum/2
  Product1/1 -> Sum/1
  Sum/1 -> Gain/1
  Demux/1 -> Product1/1
  Demux/2 -> Product1/2
  Demux/3 -> Product2/1
  Gain/1 -> A23/1
  normal(q)/1 -> Demux/1

== system Aircraft6dof_V2/Actuators - Plant /Equations Of Motion State Equations/QUAT2DCM/Subsystem5 ==
  normal(q) : Inport
  Demux : Demux
  Gain : Gain  Gain=2
  Product1 : Product  RndMeth=Zero
  Product2 : Product  RndMeth=Zero
  Sum : Sum  Inputs=|++
  A31 : Outport  VectorParamsAs1DForOutWhenUnconnected=off
  wires:
  Sum/1 -> Gain/1
  Gain/1 -> A31/1
  normal(q)/1 -> Demux/1
  Demux/3 -> Product1/2
  Demux/2 -> Product2/1
  Demux/4 -> Product2/2
  Product2/1 -> Sum/2
  Product1/1 -> Sum/1
  Demux/1 -> Product1/1

== system Aircraft6dof_V2/Actuators - Plant /Equations Of Motion State Equations/QUAT2DCM/Subsystem6 ==
  normal(q) : Inport
  Demux : Demux
  Gain : Gain  Gain=2
  Product1 : Product  RndMeth=Zero
  Product2 : Product  RndMeth=Zero
  Sum : Sum  Inputs=|-+
  A32 : Outport  VectorParamsAs1DForOutWhenUnconnected=off
  wires:
  normal(q)/1 -> Demux/1
  Gain/1 -> A32/1
  Demux/3 -> Product2/1
  Demux/2 -> Product1/2
  Demux/1 -> Product1/1
  Sum/1 -> Gain/1
  Product1/1 -> Sum/1
  Product2/1 -> Sum/2
  Demux/4 -> Product2/2

== system Aircraft6dof_V2/Actuators - Plant /Equations Of Motion State Equations/QUAT2DCM/Subsystem7 ==
  normal(q) : Inport
  Demux : Demux
  Product{,1..3} (4 alike) : Product  RndMeth=Zero
  Sum : Sum  Inputs=+-+-
  A22 : Outport  VectorParamsAs1DForOutWhenUnconnected=off
  wires:
  normal(q)/1 -> Demux/1
  Product/1 -> Sum/4
  Product1/1 -> Sum/3
  Product2/1 -> Sum/2
  Product3/1 -> Sum/1
  Demux/1 -> Product3/1, Product3/2
  Demux/2 -> Product2/1, Product2/2
  Demux/3 -> Product1/1, Product1/2
  Demux/4 -> Product/1, Product/2
  Sum/1 -> A22/1

== system Aircraft6dof_V2/Actuators - Plant /Equations Of Motion State Equations/QUAT2DCM/Subsystem8 ==
  normal(q) : Inport
  Demux : Demux
  Product{,1..3} (4 alike) : Product  RndMeth=Zero
  Sum : Sum  Inputs=+--+
  A33 : Outport  VectorParamsAs1DForOutWhenUnconnected=off
  wires:
  normal(q)/1 -> Demux/1
  Product/1 -> Sum/4
  Product1/1 -> Sum/3
  Product2/1 -> Sum/2
  Product3/1 -> Sum/1
  Demux/1 -> Product3/1, Product3/2
  Demux/2 -> Product2/1, Product2/2
  Demux/3 -> Product1/1, Product1/2
  Demux/4 -> Product/1, Product/2
  Sum/1 -> A33/1

== system Aircraft6dof_V2/Actuators - Plant /Equations Of Motion State Equations/QUAT2DCM/norm ==
  q : Inport
  Dot Product : DotProduct  OutDataTypeStr=Inherit: Inherit via internal rule
  Math Function : Math  Operator=sqrt  SignedPower=on
  e/|e| : Product  Inputs=*/  InputSameDT=on  RndMeth=Zero  SaturateOnIntegerOverflow=on  OutDataTypeStr=Inherit: Same as first input
  q/|q| : Outport  VectorParamsAs1DForOutWhenUnconnected=off
  wires:
  q/1 -> Dot Product/2, Dot Product/1, e/|e|/1
  Dot Product/1 -> Math Function/1
  Math Function/1 -> e/|e|/2
  e/|e|/1 -> q/|q|/1

== system Aircraft6dof_V2/Actuators - Plant /Equations Of Motion State Equations/Rot Dyn (Moments)/Integrate ==
  omDot : Inport
  Constant2 : Constant  Value=A8.init.InitRates
  Demux : Demux  Outputs=3
  Demux1 : Demux  Outputs=3
  Mux : Mux  Inputs=3
  P : Integrator  InitialConditionSource=external
  Q : Integrator  InitialConditionSource=external
  R : Integrator  InitialConditionSource=external
  om : Outport  VectorParamsAs1DForOutWhenUnconnected=off
  wires:
  Demux1/1 -> P/2
  P/1 -> Mux/1
  Demux/3 -> R/1
  Demux1/3 -> R/2
  Demux1/2 -> Q/2
  Q/1 -> Mux/2
  Demux/2 -> Q/1
  Mux/1 -> om/1
  Constant2/1 -> Demux1/1
  omDot/1 -> Demux/1
  Demux/1 -> P/1
  R/1 -> Mux/3

== system Aircraft6dof_V2/Actuators - Plant /Equations Of Motion State Equations/Rot Dyn (Moments)/Internal Rotational Component 1 ==
  om_B_B_BE : Inport
  om_int_dot : Inport  Port=2
  Constant1 : Constant  Value=J_int(1)
  Constant3 : Constant  Value=n_int(:,1)
  Cross Product2 : vrlib/Utilities/Cross Product
  Integrate : Subsystem
  Product2 : Product  Inputs=3
  hInt : Outport
  hIntDot : Outport  Port=2
  om_motor : Outport  Port=3
  wires:
  Product2/1 -> hIntDot/1, Integrate/1(hInt_dot)
  Cross Product2/1 -> hInt/1
  Constant1/1 -> Product2/2, Integrate/2(J)
  Constant3/1 -> Product2/3, Integrate/3(n)
  om_int_dot/1 -> Product2/1
  om_B_B_BE/1 -> Cross Product2/1
  Integrate/1(hInt) -> Cross Product2/2, om_motor/1

== system Aircraft6dof_V2/Actuators - Plant /Equations Of Motion State Equations/Rot Dyn (Moments)/Internal Rotational Component 2 ==
  om_B_B_BE : Inport
  om_int_dot : Inport  Port=2
  Constant1 : Constant  Value=J_int(1)
  Constant3 : Constant  Value=n_int(:,1)
  Cross Product2 : vrlib/Utilities/Cross Product
  Integrate : Subsystem
  Product1 : Product  Inputs=3
  Product2 : Product  Inputs=3
  Om_cross_hInt : Outport  VectorParamsAs1DForOutWhenUnconnected=off
  hIntDot : Outport  Port=2  VectorParamsAs1DForOutWhenUnconnected=off
  om_motor : Outport  Port=3  VectorParamsAs1DForOutWhenUnconnected=off
  wires:
  Product2/1 -> hIntDot/1
  Cross Product2/1 -> Om_cross_hInt/1
  Constant1/1 -> Product2/2, Product1/2
  Constant3/1 -> Product2/3, Product1/3
  om_int_dot/1 -> Integrate/1(omInt_dot), Product2/1
  om_B_B_BE/1 -> Cross Product2/1
  Integrate/1(omInt) -> om_motor/1, Product1/1
  Product1/1 -> Cross Product2/2  "hInt"

== system Aircraft6dof_V2/Actuators - Plant /Equations Of Motion State Equations/Rot Kin (Orientation) Euler/Integrate ==
  AttDot : Inport
  Constant1 : Constant  Value=InitAtt
  Demux : Demux  Outputs=3
  Demux1 : Demux  Outputs=3
  Mux : Mux  Inputs=3
  Phi : Integrator  InitialConditionSource=external
  Psi : Integrator  InitialConditionSource=external
  Theta : Integrator  InitialConditionSource=external
  Att : Outport  PortDimensions=3  VectorParamsAs1DForOutWhenUnconnected=off
  wires:
  Demux1/1 -> Phi/2
  Phi/1 -> Mux/1
  Demux/3 -> Psi/1
  Demux1/3 -> Psi/2
  Demux1/2 -> Theta/2
  Theta/1 -> Mux/2
  Demux/2 -> Theta/1
  Mux/1 -> Att/1
  Constant1/1 -> Demux1/1
  AttDot/1 -> Demux/1
  Demux/1 -> Phi/1
  Psi/1 -> Mux/3

== system Aircraft6dof_V2/Actuators - Plant /Equations Of Motion State Equations/Rot Kin (Orientation) Quaternion/QuatMult ==
  q : Inport
  r : Inport  Port=2
  Mux1 : Mux
  q0 : Subsystem
  q1 : Subsystem
  q2 : Subsystem
  q4 : Subsystem
  q*r : Outport  VectorParamsAs1DForOutWhenUnconnected=off
  wires:
  q/1 -> q4/1(q), q2/1(q), q1/1(q), q0/1(q)
  Mux1/1 -> q*r/1
  q0/1(q0) -> Mux1/1
  q4/1(q3) -> Mux1/4
  q1/1(q1) -> Mux1/2
  q2/1(q2) -> Mux1/3
  r/1 -> q4/2(r), q2/2(r), q1/2(r), q0/2(r)

== system Aircraft6dof_V2/Actuators - Plant /Equations Of Motion State Equations/Rot Kin (Orientation) Quaternion/norm1 ==
  q : Inport
  Dot Product : DotProduct  OutDataTypeStr=Inherit: Inherit via internal rule
  Math Function : Math  Operator=sqrt  SignedPower=on
  e/|e| : Product  Inputs=*/  InputSameDT=on  RndMeth=Zero  SaturateOnIntegerOverflow=on  OutDataTypeStr=Inherit: Same as first input
  q/|q| : Outport  VectorParamsAs1DForOutWhenUnconnected=off
  wires:
  e/|e|/1 -> q/|q|/1
  Math Function/1 -> e/|e|/2
  Dot Product/1 -> Math Function/1
  q/1 -> e/|e|/1, Dot Product/1, Dot Product/2

== system Aircraft6dof_V2/Actuators - Plant /Equations Of Motion State Equations/Trans Dyn (Forces)/Integrate ==
  VelDot : Inport
  Constant2 : Constant  Value=A8.init.InitVel
  Demux : Demux  Outputs=3
  Demux1 : Demux  Outputs=3
  Mux : Mux  Inputs=3
  U : Integrator  InitialConditionSource=external
  V : Integrator  InitialConditionSource=external
  W : Integrator  InitialConditionSource=external
  Vel : Outport  VectorParamsAs1DForOutWhenUnconnected=off
  wires:
  Demux1/1 -> U/2
  U/1 -> Mux/1
  Demux/3 -> W/1
  Demux1/3 -> W/2
  Demux1/2 -> V/2
  V/1 -> Mux/2
  Demux/2 -> V/1
  Mux/1 -> Vel/1
  Constant2/1 -> Demux1/1
  VelDot/1 -> Demux/1
  Demux/1 -> U/1
  W/1 -> Mux/3

== system Aircraft6dof_V2/Actuators - Plant /Equations Of Motion State Equations/Trans Kin (Spherical)/LatDot ==
  Vn : Inport
  Rearth : Inport  Port=2
  alt : Inport  Port=3
  Add : Sum
  Divide : Product  Inputs=*/
  latDot : Outport  VectorParamsAs1DForOutWhenUnconnected=off
  wires:
  Vn/1 -> Divide/1
  Add/1 -> Divide/2
  Divide/1 -> latDot/1
  alt/1 -> Add/2
  Rearth/1 -> Add/1

== system Aircraft6dof_V2/Actuators - Plant /Equations Of Motion State Equations/Trans Kin (Spherical)/LonDot ==
  Ve : Inport
  Rearth : Inport  Port=2
  alt : Inport  Port=3
  lat : Inport  Port=4
  Add1 : Sum
  Divide1 : Product  Inputs=*//
  Trigonometric Function : Trigonometry  Operator=cos
  lonDot : Outport  VectorParamsAs1DForOutWhenUnconnected=off
  wires:
  Ve/1 -> Divide1/1
  Add1/1 -> Divide1/2
  lat/1 -> Trigonometric Function/1
  Trigonometric Function/1 -> Divide1/3
  Divide1/1 -> lonDot/1
  Rearth/1 -> Add1/1
  alt/1 -> Add1/2

== system Aircraft6dof_V2/Actuators - Plant /Equations Of Motion State Equations/Trans Kin (Spherical)/wrap lon ==
  lon : Inport
  Add : Sum  Inputs=-+
  Add1 : Sum
  Compare To Constant : simulink/Logic and Bit Operations/Compare To Constant  relop=>  const=pi  OutDataTypeStr=boolean
  Compare To Constant1 : simulink/Logic and Bit Operations/Compare To Constant  relop=<=  const=-pi  OutDataTypeStr=boolean
  Constant : Constant  Value=2*pi
  Switch : Switch  Criteria=u2 > Threshold  SaturateOnIntegerOverflow=off  InputSameDT=off
  Switch1 : Switch  Criteria=u2 > Threshold  SaturateOnIntegerOverflow=off  InputSameDT=off
  -pi < lon <= pi : Outport  VectorParamsAs1DForOutWhenUnconnected=off
  wires:
  lon/1 -> Compare To Constant/1, Add/2, Switch/3
  Add/1 -> Switch/1
  Compare To Constant/1 -> Switch/2
  Compare To Constant1/1 -> Switch1/2
  Switch/1 -> Switch1/3, Add1/2, Compare To Constant1/1
  Switch1/1 -> -pi < lon <= pi/1
  Constant/1 -> Add/1, Add1/1
  Add1/1 -> Switch1/1

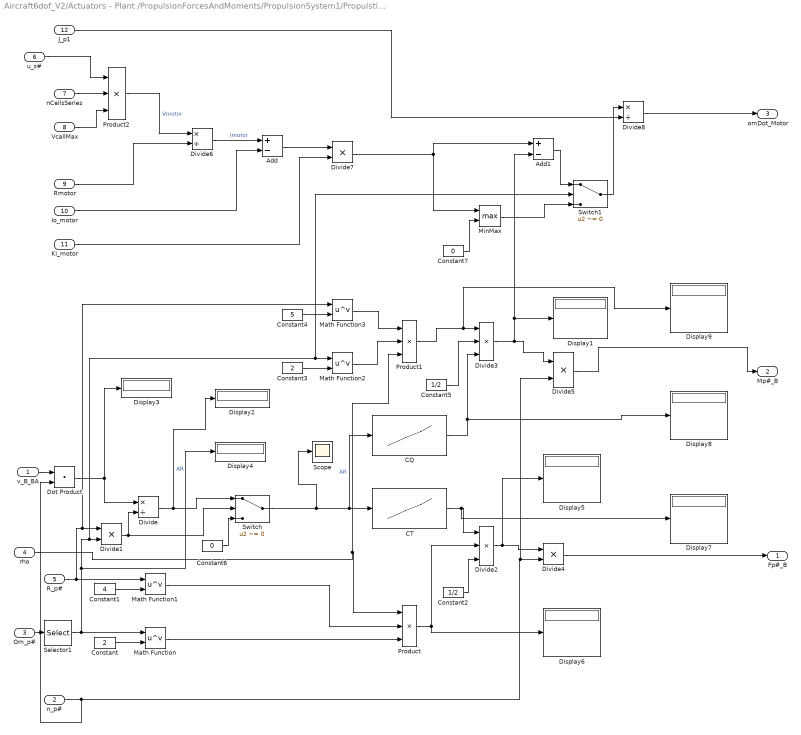
== system Aircraft6dof_V2/Actuators - Plant /PropulsionForcesAndMoments/PropulsionSystem1/PropulstionSystem# ==
  v_B_BA : Inport
  n_p# : Inport  Port=2
  Om_p# : Inport  Port=3
  rho : Inport  Port=4
  R_p# : Inport  Port=5
  u_s# : Inport  Port=6
  nCellsSeries : Inport  Port=7
  VcallMax : Inport  Port=8
  Rmotor : Inport  Port=9
  Io_motor : Inport  Port=10
  Ki_motor : Inport  Port=11
  J_p1 : Inport  Port=12
  Add : Sum  Inputs=+-
  Add1 : Sum  Inputs=+-
  CQ : Lookup_n-D  NumberOfTableDimensions=1  BreakpointsForDimension1=ARvecP1  Table=CQvecP1  ExtrapMethod=Clip  DiagnosticForOutOfRangeInput=Warning  InternalRulePriority=Speed  RndMeth=Simplest
  CT : Lookup_n-D  NumberOfTableDimensions=1  BreakpointsForDimension1=ARvecP1  Table=CTvecP1  ExtrapMethod=Clip  DiagnosticForOutOfRangeInput=Warning  InternalRulePriority=Speed  RndMeth=Simplest
  Constant : Constant  Value=2
  Constant1 : Constant  Value=4
  Constant2 : Constant  Value=1/2
  Constant3 : Constant  Value=2
  Constant4 : Constant  Value=5
  Constant5 : Constant  Value=1/2
  Constant6 : Constant  Value=0
  Constant7 : Constant  Value=0
  Display{1..9} (9 alike) : Display
  Divide : Product  Inputs=*/
  Divide{1,4..5,7} (4 alike) : Product  Inputs=**
  Divide2 : Product  Inputs=***
  Divide3 : Product  Inputs=***
  Divide6 : Product  Inputs=*/
  Divide8 : Product  Inputs=*/
  Dot Product : DotProduct  OutDataTypeStr=Inherit: Inherit via internal rule
  Math Function{,1..3} (4 alike) : Math  Operator=pow  SignedPower=on
  MinMax : MinMax  Function=max  Inputs=2
  Product : Product  Inputs=3
  Product1 : Product  Inputs=3
  Product2 : Product  Inputs=3
  Scope : Scope
      settings: ActiveDisplayYMinimum=1280  ActiveDisplayYMaximum=1293  DataLoggingVariableName=ScopeData16
  Selector1 : Selector  InputPortWidth=3  IndexOptions=Index vector (dialog)  Indices=[1]  OutputSizes=1
  Switch : Switch  Criteria=u2 ~= 0  SaturateOnIntegerOverflow=off  InputSameDT=off
  Switch1 : Switch  Criteria=u2 ~= 0  SaturateOnIntegerOverflow=off  InputSameDT=off
  Fp#_B : Outport  VectorParamsAs1DForOutWhenUnconnected=off
  Mp#_B : Outport  Port=2  VectorParamsAs1DForOutWhenUnconnected=off
  omDot_Motor : Outport  Port=3  VectorParamsAs1DForOutWhenUnconnected=off
  wires:
  Selector1/1 -> Display4/1, Switch1/2, Math Function2/1, Divide1/2, Math Function/1
  Constant/1 -> Math Function/2
  R_p#/1 -> Math Function3/1, Divide1/1, Math Function1/1
  Constant1/1 -> Math Function1/2
  rho/1 -> Product1/3, Product/1
  Math Function1/1 -> Product/2
  Math Function/1 -> Product/3
  v_B_BA/1 -> Dot Product/1
  Divide1/1 -> Divide/2, Switch/2
  Switch/1 -> Scope/1, CQ/1, CT/1  "AR"
  CT/1 -> Display7/1, Divide2/1
  Product/1 -> Divide2/2, Display6/1
  Constant2/1 -> Divide2/3
  Constant3/1 -> Math Function2/2
  Constant4/1 -> Math Function3/2
  Math Function3/1 -> Product1/1
  Math Function2/1 -> Product1/2
  Constant5/1 -> Divide3/2
  CQ/1 -> Display8/1, Divide3/3
  Product1/1 -> Display9/1, Divide3/1
  Divide2/1 -> Display5/1, Divide4/1
  n_p#/1 -> Dot Product/2, Divide5/2, Divide4/2
  Divide3/1 -> Display1/1, Add1/2, Divide5/1
  Divide4/1 -> Fp#_B/1
  Divide5/1 -> Mp#_B/1
  Divide/1 -> Display2/1, Switch/1  "AR"
  Constant6/1 -> Switch/3
  Om_p#/1 -> Selector1/1
  Dot Product/1 -> Divide/1, Display3/1
  u_s#/1 -> Product2/1
  nCellsSeries/1 -> Product2/2
  VcallMax/1 -> Product2/3
  Rmotor/1 -> Divide6/2
  Product2/1 -> Divide6/1  "Vmotor"
  Divide6/1 -> Add/1  "Imotor"
  Io_motor/1 -> Add/2
  Add/1 -> Divide7/1
  Ki_motor/1 -> Divide7/2
  Divide8/1 -> omDot_Motor/1
  J_p1/1 -> Divide8/2
  Switch1/1 -> Divide8/1
  Divide7/1 -> MinMax/1, Add1/1
  Constant7/1 -> MinMax/2
  Add1/1 -> Switch1/1
  MinMax/1 -> Switch1/3

== system Aircraft6dof_V2/Actuators - Plant /Equations Of Motion State Equations/Rot Dyn (Moments)/Internal Rotational Component 1/Integrate ==
  hInt_dot : Inport
  J : Inport  Port=2
  n : Inport  Port=3
  Constant2 : Constant  Value=A8.init.motor.om_motor_init
  Demux : Demux  Outputs=3
  Demux1 : Demux  Outputs=3
  Mux : Mux  Inputs=3
  Product1 : Product  Inputs=3
  hx : Integrator  InitialConditionSource=external
  hy : Integrator  InitialConditionSource=external
  hz : Integrator  InitialConditionSource=external
  hInt : Outport
  wires:
  Demux1/1 -> hx/2
  hx/1 -> Mux/1
  Demux/3 -> hz/1
  Demux1/3 -> hz/2
  Demux1/2 -> hy/2
  hy/1 -> Mux/2
  Demux/2 -> hy/1
  Mux/1 -> hInt/1
  Product1/1 -> Demux1/1
  hInt_dot/1 -> Demux/1
  Demux/1 -> hx/1
  hz/1 -> Mux/3
  Constant2/1 -> Product1/3
  n/1 -> Product1/2
  J/1 -> Product1/1

== system Aircraft6dof_V2/Actuators - Plant /Equations Of Motion State Equations/Rot Dyn (Moments)/Internal Rotational Component 2/Integrate ==
  omInt_dot : Inport
  Constant1 : Constant  Value=0
  Constant2 : Constant  Value=A8.init.motor.om_motor_init
  Mux : Mux  Inputs=3
  hx : Integrator  InitialConditionSource=external
  hy : Integrator  InitialConditionSource=external
  hz : Integrator  InitialConditionSource=external
  omInt : Outport  VectorParamsAs1DForOutWhenUnconnected=off
  wires:
  Constant2/1 -> hx/2
  hx/1 -> Mux/1
  Constant1/1 -> hz/1, hz/2, hy/2, hy/1
  hy/1 -> Mux/2
  Mux/1 -> omInt/1
  omInt_dot/1 -> hx/1
  hz/1 -> Mux/3

== system Aircraft6dof_V2/Actuators - Plant /Equations Of Motion State Equations/Rot Kin (Orientation) Quaternion/QuatMult/q0 ==
  q : Inport
  r : Inport  Port=2
  Demux : Demux
  Demux1 : Demux
  Product{,1..3} (4 alike) : Product  RndMeth=Zero
  Sum : Sum  Inputs=+---
  q0 : Outport  VectorParamsAs1DForOutWhenUnconnected=off
  wires:
  Product2/1 -> Sum/3
  Sum/1 -> q0/1
  Product3/1 -> Sum/4
  Product1/1 -> Sum/2
  Product/1 -> Sum/1
  Demux/4 -> Product3/1
  Demux1/4 -> Product3/2
  Demux1/3 -> Product2/2
  Demux/3 -> Product2/1
  Demux1/2 -> Product1/2
  Demux/2 -> Product1/1
  Demux1/1 -> Product/2
  Demux/1 -> Product/1
  r/1 -> Demux1/1
  q/1 -> Demux/1

== system Aircraft6dof_V2/Actuators - Plant /Equations Of Motion State Equations/Rot Kin (Orientation) Quaternion/QuatMult/q1 ==
  q : Inport
  r : Inport  Port=2
  Demux : Demux
  Demux1 : Demux
  Product{,1..3} (4 alike) : Product  RndMeth=Zero
  Sum : Sum  Inputs=+++-
  q1 : Outport  VectorParamsAs1DForOutWhenUnconnected=off
  wires:
  Demux1/3 -> Product3/2
  Demux1/4 -> Product2/2
  Demux1/1 -> Product1/2
  Demux1/2 -> Product/2
  q/1 -> Demux/1
  r/1 -> Demux1/1
  Demux/1 -> Product/1
  Demux/2 -> Product1/1
  Demux/3 -> Product2/1
  Demux/4 -> Product3/1
  Product/1 -> Sum/1
  Product1/1 -> Sum/2
  Product3/1 -> Sum/4
  Sum/1 -> q1/1
  Product2/1 -> Sum/3

== system Aircraft6dof_V2/Actuators - Plant /Equations Of Motion State Equations/Rot Kin (Orientation) Quaternion/QuatMult/q2 ==
  q : Inport
  r : Inport  Port=2
  Demux : Demux
  Demux1 : Demux
  Product{,1..3} (4 alike) : Product  RndMeth=Zero
  Sum : Sum  Inputs=+-++
  q2 : Outport  VectorParamsAs1DForOutWhenUnconnected=off
  wires:
  Demux1/2 -> Product3/2
  Demux1/1 -> Product2/2
  Demux1/4 -> Product1/2
  Demux1/3 -> Product/2
  Product2/1 -> Sum/3
  Sum/1 -> q2/1
  Product3/1 -> Sum/4
  Product1/1 -> Sum/2
  Product/1 -> Sum/1
  Demux/4 -> Product3/1
  Demux/3 -> Product2/1
  Demux/2 -> Product1/1
  r/1 -> Demux1/1
  q/1 -> Demux/1
  Demux/1 -> Product/1

== system Aircraft6dof_V2/Actuators - Plant /Equations Of Motion State Equations/Rot Kin (Orientation) Quaternion/QuatMult/q4 ==
  q : Inport
  r : Inport  Port=2
  Demux : Demux
  Demux1 : Demux
  Product{,1..3} (4 alike) : Product  RndMeth=Zero
  Sum : Sum  Inputs=++-+
  q3 : Outport  VectorParamsAs1DForOutWhenUnconnected=off
  wires:
  Demux1/4 -> Product/2
  Demux1/3 -> Product1/2
  Demux1/1 -> Product3/2
  Demux1/2 -> Product2/2
  q/1 -> Demux/1
  r/1 -> Demux1/1
  Demux/1 -> Product/1
  Demux/2 -> Product1/1
  Demux/3 -> Product2/1
  Demux/4 -> Product3/1
  Product/1 -> Sum/1
  Product1/1 -> Sum/2
  Product3/1 -> Sum/4
  Sum/1 -> q3/1
  Product2/1 -> Sum/3

== matlab function Aircraft6dof_V2/Actuators - Plant /Atmosphere Model/Standard Atmosphere - Troposphere ==
  data: h input; rho output
function rho = fcn(h)
%#codegen

temp_C = 15.04 - 0.00649 * h;
temp_K = 273.15 + temp_C;

press_NQm2 = 101.29 * (temp_K/288.08)^5.256;

rho_kgQm3 = press_NQm2 / (0.2869 *temp_K);

rho = rho_kgQm3;

== matlab function Aircraft6dof_V2/Actuators - Plant /Equations Of Motion State Equations/Rot Dyn (Moments)/inv of matrix ==
  data: u input; y output
function y = fcn(u)
%#codegen

y = inv(u);

== matlab function Aircraft6dof_V2/Actuators - Plant /Compute Wind Axes Vector/Compute Wind DCMs ==
  data: Vinf input; C_SB output; C_WB output; alpha input; beta input
function [C_SB, C_WB] = fcn(Vinf, alpha, beta)
%#codegen

C_SB = [cos(alpha)   0   sin(alpha) ;
        0           1   0         ;
        -sin(alpha)  0   cos(alpha)];
    
C_WS = [cos(beta)   sin(beta)   0 ;
        -sin(beta)  cos(beta)   0 ;
        0           0           1];
C_WB = C_WS * C_SB;

== matlab function Aircraft6dof_V2/Actuators - Plant /Equations Of Motion State Equations/Rot Kin (Orientation) Euler/MATLAB Function ==
  data: ATT input; MATRIX output
function MATRIX = EulerIntegrationMatrix(ATT)
%#codegen

phi=ATT(1);
theta=ATT(2);
psi=ATT(3);

MATRIX = [1     sin(phi)*tan(theta)   cos(phi)*tan(theta) ; 
          0     cos(phi)             -sin(phi)            ;
          0     sin(phi)/cos(theta)   cos(phi)/cos(theta)   ];

== matlab function Aircraft6dof_V2/Actuators - Plant /Equations Of Motion State Equations/MATLAB Function ==
  data: ATT input; DCM output
function DCM = ATT2DCM(ATT)
%#codegen

phi=ATT(1);
theta=ATT(2);
psi=ATT(3);

DCM = [ cos(theta)*cos(psi)                             cos(theta)*sin(psi)                            -sin(theta)          ; 
        sin(theta)*cos(psi)*sin(phi)-sin(psi)*cos(phi)  sin(theta)*sin(psi)*sin(phi)+cos(psi)*cos(phi)  cos(theta)*sin(phi) ;
        sin(theta)*cos(psi)*cos(phi)+sin(psi)*sin(phi)  sin(theta)*sin(psi)*cos(phi)-cos(psi)*sin(phi)  cos(theta)*cos(phi)   ];
